simulink model "beisp_4"  (Simulink 4.00)
settings: Solver=ode5  SolverMode=SingleTasking  StartTime=0.0  StopTime=10.0  RelTol=1e-3  AbsTol=1e-6
libraries: simulink3 x1
settings Model: LastModifiedBy=Administrator  LoadExternalInput=on  ExternalInput=A1  LimitDataPoints=off  ExtModeTrigMode=oneshot  ExtModeArmWhenConnect=off  BlockReductionOpt=off

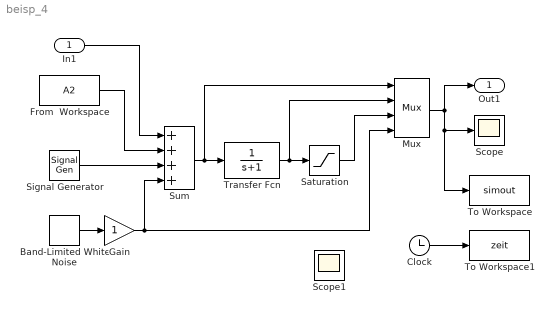
== system beisp_4 ==
  In1 : Inport  Port=1
  Band-Limited White Noise : simulink3/Sources/Band-Limited White Noise  Cov=[0.1]  Ts=0.1  seed=[23341]
  Clock : Clock
      settings: DisplayTime=off  Decimation=10
  From  Workspace : FromWorkspace  VariableName=A2  SampleTime=0  OutputAfterFinalValue=Extrapolation
  Gain : Gain  Gain=1  Multiplication=Element-wise(K.*u)  SaturateOnIntegerOverflow=on
  Mux : Mux  Inputs=4
      settings: DisplayOption=none
  Saturation : Saturate  UpperLimit=4.5  LowerLimit=-4.5  LinearizeAsGain=on
  Scope : Scope
      settings: TickLabels=on  TimeRange=auto  YMin=-5  YMax=5  SaveToWorkspace=off  SaveName=ScopeData  DataFormat=Array  LimitDataPoints=on  MaxDataPoints=5000
  Scope1 : Scope
      settings: Floating=on  TickLabels=on  TimeRange=auto  YMin=-5  YMax=5  SaveToWorkspace=off  SaveName=ScopeData  DataFormat=Array  LimitDataPoints=on  MaxDataPoints=5000
  Signal Generator : SignalGenerator  WaveForm=square  Amplitude=5  Frequency=0.15  Units=Hertz
  Sum : Sum  Inputs=++++  SaturateOnIntegerOverflow=on
  To Workspace : ToWorkspace  VariableName=simout  SampleTime=-1  SaveFormat=Array
      settings: MaxDataPoints=1000
  To Workspace1 : ToWorkspace  VariableName=zeit  SampleTime=-1  SaveFormat=Array
      settings: MaxDataPoints=1000
  Transfer Fcn : TransferFcn  Numerator=[1]  Denominator=[1 1]  Realization=auto  AbsoluteTolerance=auto
  Out1 : Outport  Port=1
  wires:
  Signal Generator/1 -> Sum/3
  From  Workspace/1 -> Sum/2
  Band-Limited White Noise/1 -> Gain/1
  Saturation/1 -> Mux/3
  Sum/1 -> Transfer Fcn/1, Mux/1
  Transfer Fcn/1 -> Saturation/1, Mux/2
  In1/1 -> Sum/1
  Gain/1 -> Sum/4, Mux/4
  Mux/1 -> Out1/1, To Workspace/1, Scope/1
  Clock/1 -> To Workspace1/1
